simulink model "Roll_Autopilot_PP"  (R2017b)
settings: Solver=FixedStepDiscrete  StartTime=0.0  StopTime=10.0  FixedStep=0.025000  RelTol=1e-3
model workspace (MAT data in the model file):
  ContractValidatorBlocksMap = containers.Map
  ContractValidatorBlocksMap.serialization.keys = {'Roll_Autopilot/Roll_Autopilot_RollAutopilotSpec/validator', 'Roll_Autopilot/Roll_Autopilot_RollAutopilotSpec1/validator'}
  ContractValidatorBlocksMap.serialization.values{1}.block = 'Roll_Autopilot/Roll_Autopilot_RollAutopilotSpec/validator'
  ContractValidatorBlocksMap.serialization.values{1}.assumePorts = 0
  ContractValidatorBlocksMap.serialization.values{1}.guaranteePorts = 6
  ContractValidatorBlocksMap.serialization.values{1}.modeBlocksPorts = 2
  ContractValidatorBlocksMap.serialization.values{1}.portHandles.Inport = [3068.00048828 3069.00048828 3070.00048828 3071.00048828 3072.00231934 3074.00231934 3078.00231934 3079.00231934]
  ContractValidatorBlocksMap.serialization.values{1}.portHandles.Outport = 3080.00231934
  ContractValidatorBlocksMap.serialization.values{1}.portHandles.Enable = []
  ContractValidatorBlocksMap.serialization.values{1}.portHandles.Trigger = []
  ContractValidatorBlocksMap.serialization.values{1}.portHandles.State = []
  ContractValidatorBlocksMap.serialization.values{1}.portHandles.LConn = []
  ContractValidatorBlocksMap.serialization.values{1}.portHandles.RConn = []
  ContractValidatorBlocksMap.serialization.values{1}.portHandles.Ifaction = []
  ContractValidatorBlocksMap.serialization.values{1}.portHandles.Reset = []
  ContractValidatorBlocksMap.serialization.values{1}.portConnectivity(1).Type = '1'
  ContractValidatorBlocksMap.serialization.values{1}.portConnectivity(1).Position = [31840 -150]
  ContractValidatorBlocksMap.serialization.values{1}.portConnectivity(1).SrcBlock = 1525.00219727
  ContractValidatorBlocksMap.serialization.values{1}.portConnectivity(1).SrcPort = 0
  ContractValidatorBlocksMap.serialization.values{1}.portConnectivity(1).DstBlock = []
  ContractValidatorBlocksMap.serialization.values{1}.portConnectivity(1).DstPort = []
  ContractValidatorBlocksMap.serialization.values{1}.portConnectivity(2).Type = '2'
  ContractValidatorBlocksMap.serialization.values{1}.portConnectivity(2).Position = [31840 -85]
  ContractValidatorBlocksMap.serialization.values{1}.portConnectivity(2).SrcBlock = 1545.00048828
  ContractValidatorBlocksMap.serialization.values{1}.portConnectivity(2).SrcPort = 0
  ContractValidatorBlocksMap.serialization.values{1}.portConnectivity(2).DstBlock = []
  ContractValidatorBlocksMap.serialization.values{1}.portConnectivity(2).DstPort = []
  ContractValidatorBlocksMap.serialization.values{1}.portConnectivity(3).Type = '3'
  ContractValidatorBlocksMap.serialization.values{1}.portConnectivity(3).Position = [31840 -20]
  ContractValidatorBlocksMap.serialization.values{1}.portConnectivity(3).SrcBlock = 1541.00048828
  ContractValidatorBlocksMap.serialization.values{1}.portConnectivity(3).SrcPort = 0
  ContractValidatorBlocksMap.serialization.values{1}.portConnectivity(3).DstBlock = []
  ContractValidatorBlocksMap.serialization.values{1}.portConnectivity(3).DstPort = []
  ContractValidatorBlocksMap.serialization.values{1}.portConnectivity(4).Type = '4'
  ContractValidatorBlocksMap.serialization.values{1}.portConnectivity(4).Position = [31840 45]
  ContractValidatorBlocksMap.serialization.values{1}.portConnectivity(4).SrcBlock = 1537.00048828
  ContractValidatorBlocksMap.serialization.values{1}.portConnectivity(4).SrcPort = 0
  ContractValidatorBlocksMap.serialization.values{1}.portConnectivity(4).DstBlock = []
  ContractValidatorBlocksMap.serialization.values{1}.portConnectivity(4).DstPort = []
  ContractValidatorBlocksMap.serialization.values{1}.portConnectivity(5).Type = '5'
  ContractValidatorBlocksMap.serialization.values{1}.portConnectivity(5).Position = [31840 110]
  ContractValidatorBlocksMap.serialization.values{1}.portConnectivity(5).SrcBlock = 1533.00219727
  ContractValidatorBlocksMap.serialization.values{1}.portConnectivity(5).SrcPort = 0
  ContractValidatorBlocksMap.serialization.values{1}.portConnectivity(5).DstBlock = []
  ContractValidatorBlocksMap.serialization.values{1}.portConnectivity(5).DstPort = []
  ContractValidatorBlocksMap.serialization.values{1}.portConnectivity(6).Type = '6'
  ContractValidatorBlocksMap.serialization.values{1}.portConnectivity(6).Position = [31840 175]
  ContractValidatorBlocksMap.serialization.values{1}.portConnectivity(6).SrcBlock = 1549.00048828
  ContractValidatorBlocksMap.serialization.values{1}.portConnectivity(6).SrcPort = 0
  ContractValidatorBlocksMap.serialization.values{1}.portConnectivity(6).DstBlock = []
  ContractValidatorBlocksMap.serialization.values{1}.portConnectivity(6).DstPort = []
  ContractValidatorBlocksMap.serialization.values{1}.portConnectivity(7).Type = '7'
  ContractValidatorBlocksMap.serialization.values{1}.portConnectivity(7).Position = [31840 240]
  ContractValidatorBlocksMap.serialization.values{1}.portConnectivity(7).SrcBlock = 2047.00048828
  ContractValidatorBlocksMap.serialization.values{1}.portConnectivity(7).SrcPort = 0
  ContractValidatorBlocksMap.serialization.values{1}.portConnectivity(7).DstBlock = []
  ContractValidatorBlocksMap.serialization.values{1}.portConnectivity(7).DstPort = []
  ContractValidatorBlocksMap.serialization.values{1}.portConnectivity(8).Type = '8'
  ContractValidatorBlocksMap.serialization.values{1}.portConnectivity(8).Position = [31840 305]
  ContractValidatorBlocksMap.serialization.values{1}.portConnectivity(8).SrcBlock = 2007.00048828
  ContractValidatorBlocksMap.serialization.values{1}.portConnectivity(8).SrcPort = 0
  ContractValidatorBlocksMap.serialization.values{1}.portConnectivity(8).DstBlock = []
  ContractValidatorBlocksMap.serialization.values{1}.portConnectivity(8).DstPort = []
  ContractValidatorBlocksMap.serialization.values{1}.portConnectivity(9).Type = '1'
  ContractValidatorBlocksMap.serialization.values{1}.portConnectivity(9).Position = [31975 80]
  ContractValidatorBlocksMap.serialization.values{1}.portConnectivity(9).SrcBlock = []
  ContractValidatorBlocksMap.serialization.values{1}.portConnectivity(9).SrcPort = []
  ContractValidatorBlocksMap.serialization.values{1}.portConnectivity(9).DstBlock = 2349.00292969
  ContractValidatorBlocksMap.serialization.values{1}.portConnectivity(9).DstPort = 0
  ContractValidatorBlocksMap.serialization.values{2}.block = 'Roll_Autopilot/Roll_Autopilot_RollAutopilotSpec1/validator'
  ContractValidatorBlocksMap.serialization.values{2}.assumePorts = 0
  ContractValidatorBlocksMap.serialization.values{2}.guaranteePorts = 6
  ContractValidatorBlocksMap.serialization.values{2}.modeBlocksPorts = 2
  ContractValidatorBlocksMap.serialization.values{2}.portHandles.Inport = [7302.00048828 7304.00048828 7306.00048828 7308.00048828 7313.00048828 7319.00048828 7322.00048828 7326.00048828]
  ContractValidatorBlocksMap.serialization.values{2}.portHandles.Outport = 7710.00048828
  ContractValidatorBlocksMap.serialization.values{2}.portHandles.Enable = []
  ContractValidatorBlocksMap.serialization.values{2}.portHandles.Trigger = []
  ContractValidatorBlocksMap.serialization.values{2}.portHandles.State = []
  ContractValidatorBlocksMap.serialization.values{2}.portHandles.LConn = []
  ContractValidatorBlocksMap.serialization.values{2}.portHandles.RConn = []
  ContractValidatorBlocksMap.serialization.values{2}.portHandles.Ifaction = []
  ContractValidatorBlocksMap.serialization.values{2}.portHandles.Reset = []
  ContractValidatorBlocksMap.serialization.values{2}.portConnectivity(1).Type = '1'
  ContractValidatorBlocksMap.serialization.values{2}.portConnectivity(1).Position = [74140 -150]
  ContractValidatorBlocksMap.serialization.values{2}.portConnectivity(1).SrcBlock = 3094.00231934
  ContractValidatorBlocksMap.serialization.values{2}.portConnectivity(1).SrcPort = 0
  ContractValidatorBlocksMap.serialization.values{2}.portConnectivity(1).DstBlock = []
  ContractValidatorBlocksMap.serialization.values{2}.portConnectivity(1).DstPort = []
  ContractValidatorBlocksMap.serialization.values{2}.portConnectivity(2).Type = '2'
  ContractValidatorBlocksMap.serialization.values{2}.portConnectivity(2).Position = [74140 -85]
  ContractValidatorBlocksMap.serialization.values{2}.portConnectivity(2).SrcBlock = 3118.00231934
  ContractValidatorBlocksMap.serialization.values{2}.portConnectivity(2).SrcPort = 0
  ContractValidatorBlocksMap.serialization.values{2}.portConnectivity(2).DstBlock = []
  ContractValidatorBlocksMap.serialization.values{2}.portConnectivity(2).DstPort = []
  ContractValidatorBlocksMap.serialization.values{2}.portConnectivity(3).Type = '3'
  ContractValidatorBlocksMap.serialization.values{2}.portConnectivity(3).Position = [74140 -20]
  ContractValidatorBlocksMap.serialization.values{2}.portConnectivity(3).SrcBlock = 3110.00231934
  ContractValidatorBlocksMap.serialization.values{2}.portConnectivity(3).SrcPort = 0
  ContractValidatorBlocksMap.serialization.values{2}.portConnectivity(3).DstBlock = []
  ContractValidatorBlocksMap.serialization.values{2}.portConnectivity(3).DstPort = []
  ContractValidatorBlocksMap.serialization.values{2}.portConnectivity(4).Type = '4'
  ContractValidatorBlocksMap.serialization.values{2}.portConnectivity(4).Position = [74140 45]
  ContractValidatorBlocksMap.serialization.values{2}.portConnectivity(4).SrcBlock = 3106.00231934
  ContractValidatorBlocksMap.serialization.values{2}.portConnectivity(4).SrcPort = 0
  ContractValidatorBlocksMap.serialization.values{2}.portConnectivity(4).DstBlock = []
  ContractValidatorBlocksMap.serialization.values{2}.portConnectivity(4).DstPort = []
  ContractValidatorBlocksMap.serialization.values{2}.portConnectivity(5).Type = '5'
  ContractValidatorBlocksMap.serialization.values{2}.portConnectivity(5).Position = [74140 110]
  ContractValidatorBlocksMap.serialization.values{2}.portConnectivity(5).SrcBlock = 3098.00231934
  ContractValidatorBlocksMap.serialization.values{2}.portConnectivity(5).SrcPort = 0
  ContractValidatorBlocksMap.serialization.values{2}.portConnectivity(5).DstBlock = []
  ContractValidatorBlocksMap.serialization.values{2}.portConnectivity(5).DstPort = []
  ContractValidatorBlocksMap.serialization.values{2}.portConnectivity(6).Type = '6'
  ContractValidatorBlocksMap.serialization.values{2}.portConnectivity(6).Position = [74140 175]
  ContractValidatorBlocksMap.serialization.values{2}.portConnectivity(6).SrcBlock = 3122.00231934
  ContractValidatorBlocksMap.serialization.values{2}.portConnectivity(6).SrcPort = 0
  ContractValidatorBlocksMap.serialization.values{2}.portConnectivity(6).DstBlock = []
  ContractValidatorBlocksMap.serialization.values{2}.portConnectivity(6).DstPort = []
  ContractValidatorBlocksMap.serialization.values{2}.portConnectivity(7).Type = '7'
  ContractValidatorBlocksMap.serialization.values{2}.portConnectivity(7).Position = [74140 240]
  ContractValidatorBlocksMap.serialization.values{2}.portConnectivity(7).SrcBlock = 3628.00061035
  ContractValidatorBlocksMap.serialization.values{2}.portConnectivity(7).SrcPort = 0
  ContractValidatorBlocksMap.serialization.values{2}.portConnectivity(7).DstBlock = []
  ContractValidatorBlocksMap.serialization.values{2}.portConnectivity(7).DstPort = []
  ContractValidatorBlocksMap.serialization.values{2}.portConnectivity(8).Type = '8'
  ContractValidatorBlocksMap.serialization.values{2}.portConnectivity(8).Position = [74140 305]
  ContractValidatorBlocksMap.serialization.values{2}.portConnectivity(8).SrcBlock = 3594.00061035
  ContractValidatorBlocksMap.serialization.values{2}.portConnectivity(8).SrcPort = 0
  ContractValidatorBlocksMap.serialization.values{2}.portConnectivity(8).DstBlock = []
  ContractValidatorBlocksMap.serialization.values{2}.portConnectivity(8).DstPort = []
  ContractValidatorBlocksMap.serialization.values{2}.portConnectivity(9).Type = '1'
  ContractValidatorBlocksMap.serialization.values{2}.portConnectivity(9).Position = [74275 80]
  ContractValidatorBlocksMap.serialization.values{2}.portConnectivity(9).SrcBlock = []
  ContractValidatorBlocksMap.serialization.values{2}.portConnectivity(9).SrcPort = []
  ContractValidatorBlocksMap.serialization.values{2}.portConnectivity(9).DstBlock = 4161.00061035
  ContractValidatorBlocksMap.serialization.values{2}.portConnectivity(9).DstPort = 0
  ContractValidatorBlocksMap.serialization.uniformity = 0
  ContractValidatorBlocksMap.serialization.keyType = 'char'
  ContractValidatorBlocksMap.serialization.valueType = 'any'
  already_pp = 1
  compositionalMap.analysisNames = {'Roll_Autopilot_PP/Roll_Autopilot', 'Roll_Autopilot_PP/Roll_Autopilot (one mode active)', '_floor'}
  compositionalMap.compositionalOptions = {{'', ''}, {''}, {''}}
  compositionalMap.selectedOptions = [2 1 1]
  maskControlsMap = containers.Map
  maskControlsMap.serialization.keys = {'Roll_Autopilot_PP/Roll_Autopilot_RollAutopilotSpec1/AP_minus_003A', 'Roll_Autopilot_PP/Roll_Autopilot_RollAutopilotSpec1/AP_minus_003B', 'Roll_Autopilot_PP/Roll_Autopilot_RollAutopilotSpec1/AP_minus_003C', 'Roll_Autopilot_PP/Roll_Autopilot_RollAutopilotSpec1/validator'}
  maskControlsMap.serialization.values = {{'Display_counter_example_as_signals', 'Display_counter_example_as_tables', 'Display_counter_example_as_HTML_tables', 'Generate_an_outer_model_for_the_counter_example', 'Generate_an_inner_model_for_the_counter_example'}, {'Display_counter_example_as_signals', 'Display_counter_example_as_tables', 'Display_counter_example_as_HTML_tables', 'Generate_an_outer_model_for_the_counter_example', 'Generate_an_inner_model_for_the_counter_example'}, {'Display_counter_example_as_signals', 'Display_counter_example_as_tables', 'Display_counter_example_as_HTML_tables', 'Generate_an_outer_model_for_the_counter_example', 'Generate_an_inner_model_for_the_counter_example'}, {'Display_counter_example_as_signals', 'Display_counter_example_as_tables', 'Display_counter_example_as_HTML_tables', 'Generate_an_outer_model_for_the_counter_example', 'Generate_an_inner_model_for_the_counter_example'}}
  maskControlsMap.serialization.uniformity = 0
  maskControlsMap.serialization.keyType = 'char'
  maskControlsMap.serialization.valueType = 'any'
  nodeNameToBlockNameMap : containers.Map (value not decoded)
  verificationResults : struct (value not decoded)
undefined symbols (not defined in the file): contractAfterSimulation, contractBeforeSimulation, ContractBlock, ContractEnsureBlock, ContractGuaranteeBlock, ContractModeBlock, ContractRequireBlock, ContractValidatorBlock, pp_lib, saturation, saveValidatorParameters, slcm, Ts
(part 1 of 3)
settings Model: Creator=hbourbou  LastModifiedBy=hbourbou
settings DataIOCC: ReturnWorkspaceOutputs=on
settings DebuggingCC: AlgebraicLoopMsg=error  ArtificialAlgebraicLoopMsg=error  SingleTaskRateTransMsg=error
settings SFSimCC: SimUseLocalCustomCode=on
settings RTWCC: RTWUseLocalCustomCode=on

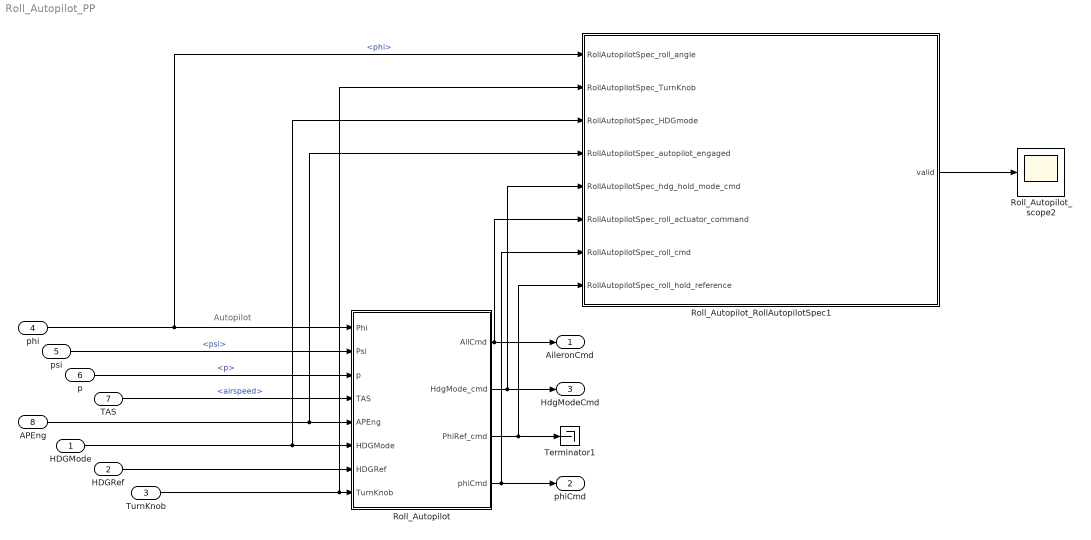
== system Roll_Autopilot_PP ==
  note: Autopilot
  HDGMode : Inport  OutMin=0  OutMax=1  OutDataTypeStr=boolean  PortDimensions=1
  HDGRef : Inport  Port=2  OutMin=-180  OutMax=180  OutDataTypeStr=double  PortDimensions=1
  TurnKnob : Inport  Port=3  OutMin=-45  OutMax=45  OutDataTypeStr=double  PortDimensions=1
  phi : Inport  Port=4
  psi : Inport  Port=5
  p : Inport  Port=6
  TAS : Inport  Port=7
  APEng : Inport  Port=8  OutDataTypeStr=boolean
  Roll_Autopilot : Subsystem  TreatAsAtomicUnit=on
  Roll_Autopilot_RollAutopilotSpec1 : Subsystem  TreatAsAtomicUnit=on  mask(ContractBlock){ContractBlockType=ContractBlock}
      mask init:
      | set_param(gcb, 'LinkStatus', 'none');
      mask DialogControl DescTextVar Prompt: Contract block
      mask Display:
      | text(0.5, 0.5, '{\bf\fontsize{20}Contract}', 'hor', 'center', 'texmode','on');
      | blocks = find_system(gcb, 'LookUnderMasks','all', 'SearchDepth',1,'BlockType','Inport');
      | for i = 1 : length(blocks)
      |     blockName = get_param(blocks(i), 'Name');
      |     [path, blockName] = fileparts(char(blockName));
      |     port_label('input', i, blockName);
      | end
      | 
      | blocks = find_system(gcb, 'LookUnderMasks','all', 'SearchDepth',1,'BlockType','Outport');
      | for i = 1 : length(blocks)
      |     blockName = get_param(blocks(i), 'Name');
      |     [path, blockName] = fileparts(char(blockName));
      |     port_label('output', i, blockName);
      | end
  Roll_Autopilot_scope2 : Scope
  Terminator1 : Terminator
  AileronCmd : Outport  OutDataTypeStr=double  PortDimensions=1  SampleTime=[0.025000000000000001,0]  VectorParamsAs1DForOutWhenUnconnected=off
  phiCmd : Outport  Port=2  VectorParamsAs1DForOutWhenUnconnected=off
  HdgModeCmd : Outport  Port=3  VectorParamsAs1DForOutWhenUnconnected=off
  wires:
  APEng/1 -> Roll_Autopilot_RollAutopilotSpec1/4(RollAutopilotSpec_autopilot_engaged), Roll_Autopilot/5(APEng)
  TAS/1 -> Roll_Autopilot/4(TAS)  "<airspeed>"
  Roll_Autopilot/2(HdgMode_cmd) -> Roll_Autopilot_RollAutopilotSpec1/5(RollAutopilotSpec_hdg_hold_mode_cmd), HdgModeCmd/1
  TurnKnob/1 -> Roll_Autopilot_RollAutopilotSpec1/2(RollAutopilotSpec_TurnKnob), Roll_Autopilot/8(TurnKnob)
  phi/1 -> Roll_Autopilot_RollAutopilotSpec1/1(RollAutopilotSpec_roll_angle), Roll_Autopilot/1(Phi)  "<phi>"
  HDGMode/1 -> Roll_Autopilot_RollAutopilotSpec1/3(RollAutopilotSpec_HDGmode), Roll_Autopilot/6(HDGMode)
  HDGRef/1 -> Roll_Autopilot/7(HDGRef)
  p/1 -> Roll_Autopilot/3(p)  "<p>"
  Roll_Autopilot/1(AilCmd) -> Roll_Autopilot_RollAutopilotSpec1/6(RollAutopilotSpec_roll_actuator_command), AileronCmd/1
  psi/1 -> Roll_Autopilot/2(Psi)  "<psi>"
  Roll_Autopilot/4(phiCmd) -> Roll_Autopilot_RollAutopilotSpec1/7(RollAutopilotSpec_roll_cmd), phiCmd/1
  Roll_Autopilot/3(PhiRef_cmd) -> Roll_Autopilot_RollAutopilotSpec1/8(RollAutopilotSpec_roll_hold_reference), Terminator1/1
  Roll_Autopilot_RollAutopilotSpec1/1(valid) -> Roll_Autopilot_scope2/1

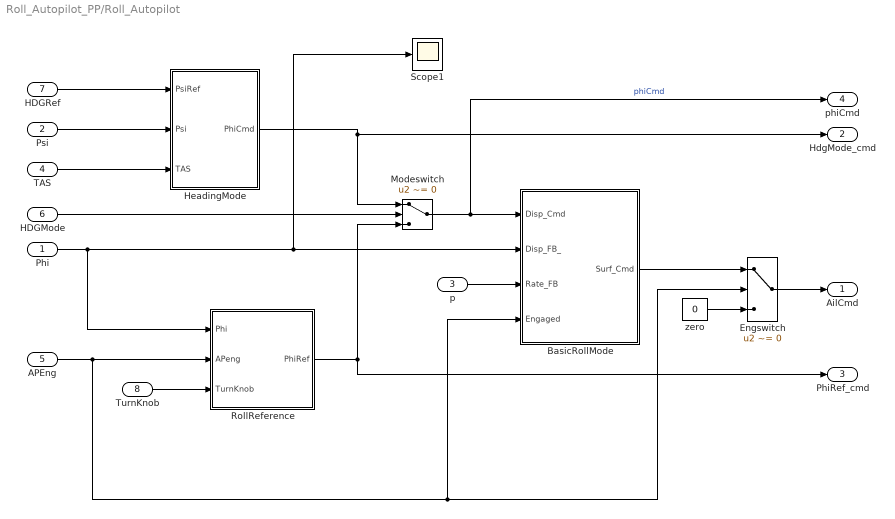
== system Roll_Autopilot_PP/Roll_Autopilot ==
  Phi : Inport  OutMin=-180  OutMax=180  OutDataTypeStr=double  PortDimensions=1  SampleTime=1/40  Interpolate=off
  Psi : Inport  Port=2  OutMin=-180  OutMax=180  OutDataTypeStr=double  PortDimensions=1  SampleTime=1/40  Interpolate=off
  p : Inport  Port=3  OutMin=-180  OutMax=180  OutDataTypeStr=double  PortDimensions=1  Interpolate=off
  TAS : Inport  Port=4  OutMin=0  OutMax=1000  OutDataTypeStr=double  PortDimensions=1  SampleTime=1/40  Interpolate=off
  APEng : Inport  Port=5  OutDataTypeStr=boolean  PortDimensions=1  SampleTime=1/40  Interpolate=off
  HDGMode : Inport  Port=6  OutDataTypeStr=boolean  PortDimensions=1  SampleTime=1/40  Interpolate=off
  HDGRef : Inport  Port=7  OutMin=-180  OutMax=180  OutDataTypeStr=double  PortDimensions=1  SampleTime=1/40  Interpolate=off
  TurnKnob : Inport  Port=8  OutMin=-45  OutMax=45  OutDataTypeStr=double  PortDimensions=1  SampleTime=1/40  Interpolate=off
  BasicRollMode : Subsystem  TreatAsAtomicUnit=on
  Engswitch : Switch  Criteria=u2 ~= 0
  HeadingMode : Subsystem  TreatAsAtomicUnit=on
  Modeswitch : Switch  Criteria=u2 ~= 0
  RollReference : Subsystem  TreatAsAtomicUnit=on
      settings: RTWSystemCode=Inline
  Scope1 : Scope
  zero : Constant  Value=0  OutDataTypeStr=double
  AilCmd : Outport  OutDataTypeStr=double  PortDimensions=1  SampleTime=1/40  VectorParamsAs1DForOutWhenUnconnected=off
  HdgMode_cmd : Outport  Port=2  VectorParamsAs1DForOutWhenUnconnected=off
  PhiRef_cmd : Outport  Port=3  VectorParamsAs1DForOutWhenUnconnected=off
  phiCmd : Outport  Port=4  VectorParamsAs1DForOutWhenUnconnected=off
  wires:
  HDGRef/1 -> HeadingMode/1(PsiRef)
  HeadingMode/1(PhiCmd) -> HdgMode_cmd/1, Modeswitch/1
  Modeswitch/1 -> phiCmd/1, BasicRollMode/1(Disp_Cmd)  "phiCmd"
  Engswitch/1 -> AilCmd/1
  APEng/1 -> RollReference/2(APeng), BasicRollMode/4(Engaged), Engswitch/2
  TAS/1 -> HeadingMode/3(TAS)
  HDGMode/1 -> Modeswitch/2
  RollReference/1(PhiRef) -> Modeswitch/3, PhiRef_cmd/1
  TurnKnob/1 -> RollReference/3(TurnKnob)
  zero/1 -> Engswitch/3
  p/1 -> BasicRollMode/3(Rate_FB)
  Phi/1 -> Scope1/1, BasicRollMode/2(Disp_FB_), RollReference/1(Phi)
  Psi/1 -> HeadingMode/2(Psi)
  BasicRollMode/1(Surf_Cmd) -> Engswitch/1
